simulink model "simul1"  (R2017a)
settings: Solver=VariableStepAuto  StartTime=0.0  StopTime=10.0  RelTol=1e-3
libraries: simulink x1
settings Model: Creator=Yajur  LastModifiedBy=Yajur

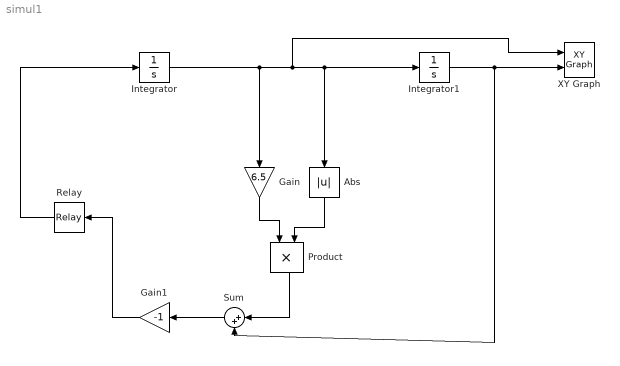
== system simul1 ==
  Abs : Abs
  Gain : Gain  Gain=6.5
  Gain1 : Gain  Gain=-1
  Integrator : Integrator  InitialCondition=-2
  Integrator1 : Integrator  InitialCondition=2
  Product : Product
  Relay : Relay
  Sum : Sum  Inputs=|++
  XY Graph : simulink/Sinks/XY Graph  xmin=-1  xmax=1  ymin=-1  ymax=1  st=-1
  wires:
  Integrator/1 -> Gain/1, XY Graph/1, Abs/1, Integrator1/1
  Gain/1 -> Product/1
  Abs/1 -> Product/2
  Integrator1/1 -> Sum/2, XY Graph/2
  Product/1 -> Sum/1
  Sum/1 -> Gain1/1
  Gain1/1 -> Relay/1
  Relay/1 -> Integrator/1
